simulink model "PID0"  (R2020b)
settings: Solver=VariableStepAuto  StartTime=0.0  StopTime=0.2  RelTol=1e-3
model workspace (MAT data in the model file):
  kd = Simulink.Parameter
  kd.Value = 50
  kd.DataType = 'auto'
  kd.Dimensions = [1 1]
  ki = Simulink.Parameter
  ki.Value = 22000
  ki.DataType = 'auto'
  ki.Dimensions = [1 1]
  kp = Simulink.Parameter
  kp.Value = 22000
  kp.DataType = 'auto'
  kp.Dimensions = [1 1]
settings Model: Creator=HP  LastModifiedBy=HP
settings DataIOCC: SaveOutput=off  SaveTime=off

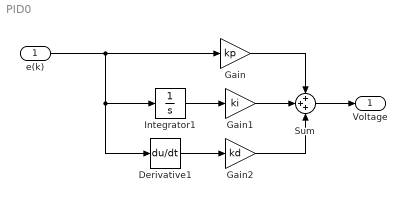
== system PID0 ==
  e(k) : Inport  OutDataTypeStr=double  PortDimensions=1  SampleTime=0
  Derivative1 : Derivative
  Gain : Gain  Gain=kp
  Gain1 : Gain  Gain=ki
  Gain2 : Gain  Gain=kd
  Integrator1 : Integrator
  Sum : Sum  Inputs=+++
  Voltage : Outport  OutDataTypeStr=double  PortDimensions=1  SampleTime=0
  wires:
  Gain2/1 -> Sum/3
  e(k)/1 -> Gain/1, Integrator1/1, Derivative1/1
  Gain/1 -> Sum/1
  Gain1/1 -> Sum/2
  Sum/1 -> Voltage/1
  Integrator1/1 -> Gain1/1
  Derivative1/1 -> Gain2/1
